simulink model "LowPassFilter2p1"  (R2019b)
settings: Solver=VariableStepAuto  StartTime=0.0  StopTime=10.0  RelTol=1e-3
settings Model: Creator=a4327  LastModifiedBy=a4327

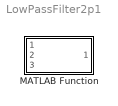
== system LowPassFilter2p1 ==
  MATLAB Function : MATLAB Function  TreatAsAtomicUnit=on

== matlab function LowPassFilter2p1/MATLAB Function ==
  data: sample input; sample_out output; sample_freq input; cutoff_freq input
function sample_out = LowPassFilter2p(sample,sample_freq,  cutoff_freq)

persistent params
    if isempty(params)
    params=compute_params( sample_freq,  cutoff_freq);
    end
sample_out= DigitalBiquadFilter_apply(sample, params);
